simulink model "power_upfc_gto48p_mdl"  (Simulink 8.3)
settings: Solver=FixedStepDiscrete  SolverMode=SingleTasking  StartTime=0.0  StopTime=0.8  FixedStep=Ts  RelTol=1e-3
PreLoadFcn:
  | Ts=1/512/60;
undefined symbols (not defined in the file or in its folder): DiscIntNeverNeededParam
libraries: powerlib x54, powerlib_meascontrol x30, simulink_extras x2, simulink x1
(part 1 of 7)
Description:
  | Copyright 2008-2014 The MathWorks, Inc.
settings Model: Creator=MathWorks  LastModifiedBy=snt  ExtModeTrigMode=oneshot  ExtModeArmWhenConnect=off  ExtModeAutoUpdateStatusClock=off
settings DataIOCC: InitialState=xInitial_upfc  LimitDataPoints=off  SaveFinalState=on  SaveFormat=Structure  SaveOutput=off  SaveTime=off  SignalLoggingName=sigsOut
settings OptimizationCC: BlockReduction=off  BooleanDataType=off  ExpressionDepthLimit=2147483647  InitFltsAndDblsToZero=on  EfficientMapNaN2IntZero=off
settings DebuggingCC: SignalResolutionControl=TryResolveAllWithWarning  SolverPrmCheckMsg=none  MultiTaskDSMMsg=warning  MultiTaskCondExecSysMsg=none  FcnCallInpInsideContextMsg=UseLocalSettings
settings HardwareCC: TargetEndianess=LittleEndian  TargetHWDeviceType=MATLAB Host  ProdEqTarget=off
settings RTWCC: SystemTargetFile=accel.tlc  TemplateMakefile=accel_default_tmf  ProcessScript=accel_make_rtw_hook  IncludeERTFirstTime=on
settings STFCustomTargetCC: GeneratePreprocessorConditionals=Disable all  MATLABClassNameForMDSCustomization=Simulink.SoftwareTarget.TargetSpecificTriggerConfigurationBase  SystemTargetFile=accel.tlc

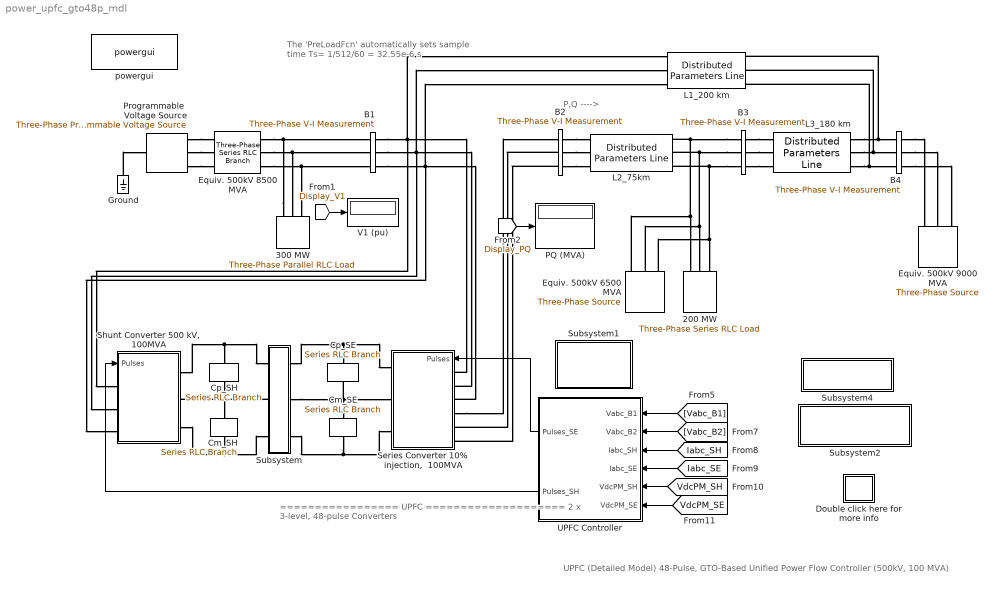
== system power_upfc_gto48p_mdl ==
  note: ================= UPFC ====================
      | 2 x   3-level, 48-pulse Converters
  note: The 'PreLoadFcn' automatically sets
      |  sample time Ts= 1/512/60 = 32.55e-6 s
  note: P,Q
      | ---->
  note: UPFC (Detailed Model)
      | 48-Pulse, GTO-Based Unified Power Flow Controller (500kV, 100 MVA)
  200 MW : powerlib/Elements/Three-Phase Series RLC Load  LConnTagsString=A|B|C  Configuration=Y (grounded)  NominalVoltage=500e3  NominalFrequency=60  ActivePower=200e6  InductivePower=0  CapacitivePower=0  Measurements=None  LoadType=constant Z
  300 MW : powerlib/Elements/Three-Phase Parallel RLC Load  LConnTagsString=A|B|C  Configuration=Y (grounded)  NominalVoltage=500e3  NominalFrequency=60  ActivePower=300e6  InductivePower=0  CapacitivePower=0  Measurements=None  LoadType=constant Z
  B1 : powerlib/Measurements/Three-Phase V-I Measurement  VoltageMeasurement=phase-to-ground  SetLabelV=on  LabelV=Vabc_B1  Vpu=on  VpuLL=off  CurrentMeasurement=yes  SetLabelI=on  LabelI=Iabc_B1  Ipu=on  Pbase=100e6  Vbase=500e3  OutputType=Magnitude  PhasorSimulation=off  PSBequivalent=0
  B2 : powerlib/Measurements/Three-Phase V-I Measurement  VoltageMeasurement=phase-to-ground  SetLabelV=on  LabelV=Vabc_B2  Vpu=on  VpuLL=off  CurrentMeasurement=yes  SetLabelI=on  LabelI=Iabc_B2  Ipu=on  Pbase=100e6  Vbase=500e3  OutputType=Magnitude  PhasorSimulation=off  PSBequivalent=0
  B3 : powerlib/Measurements/Three-Phase V-I Measurement  VoltageMeasurement=phase-to-ground  SetLabelV=on  LabelV=Vabc_B3  Vpu=on  VpuLL=off  CurrentMeasurement=yes  SetLabelI=on  LabelI=Iabc_B3  Ipu=on  Pbase=100e6  Vbase=500e3  OutputType=Magnitude  PhasorSimulation=off  PSBequivalent=0
  B4 : powerlib/Measurements/Three-Phase V-I Measurement  VoltageMeasurement=phase-to-ground  SetLabelV=on  LabelV=Vabc_B4  Vpu=on  VpuLL=off  CurrentMeasurement=no  SetLabelI=on  LabelI=Iabc_B4  Ipu=on  Pbase=100e6  Vbase=500e3  OutputType=Magnitude  PhasorSimulation=off  PSBequivalent=0
  Cm_SE : powerlib/Elements/Series RLC Branch  LConnTagsString=__new0  RConnTagsString=__new0  BranchType=C  Resistance=1.0  Inductance=1.0  SetiL0=off  InitialCurrent=0  Capacitance=2500e-6  Setx0=off  InitialVoltage=0  Measurements=Branch voltage
  Cm_SH : powerlib/Elements/Series RLC Branch  LConnTagsString=__new0  RConnTagsString=__new0  BranchType=C  Resistance=1.0  Inductance=1.0  SetiL0=off  InitialCurrent=0  Capacitance=2500e-6  Setx0=off  InitialVoltage=0  Measurements=Branch voltage
  Cp_SE : powerlib/Elements/Series RLC Branch  LConnTagsString=__new0  RConnTagsString=__new0  BranchType=C  Resistance=1.0  Inductance=1.0  SetiL0=off  InitialCurrent=0  Capacitance=2500e-6  Setx0=off  InitialVoltage=0  Measurements=Branch voltage
  Cp_SH : powerlib/Elements/Series RLC Branch  LConnTagsString=__new0  RConnTagsString=__new0  BranchType=C  Resistance=1.0  Inductance=1.0  SetiL0=off  InitialCurrent=0  Capacitance=2500e-6  Setx0=off  InitialVoltage=0  Measurements=Branch voltage
  Double click here for more info : Subsystem
      settings: OpenFcn=showdemo(bdroot(gcb))
      mask Display: disp('?')
  Equiv. 500kV 6500 MVA : powerlib/Electrical Sources/Three-Phase Source  Voltage=500e3*1.00  PhaseAngle=9.2-20  Frequency=60  InternalConnection=Yg  SpecifyImpedance=on  Resistance=0.8929  Inductance=16.58e-3  ShortCircuitLevel=6500e6  BaseVoltage=500e3  XRratio=8  BusType=swing  Pref=0  Qref=0  Qmin=-inf  Qmax=inf
  "Equiv. 500kV 8500 MVA " : powerlib/Elements/Three-Phase Series RLC Branch  LConnTagsString=A|B|C  RConnTagsString=A|B|C  BranchType=RL  Resistance=500e3^2/8500e6/10  Inductance=500e3^2/8500e6/(2*pi*60)  Capacitance=1.0  Measurements=None
  Equiv. 500kV 9000 MVA : powerlib/Electrical Sources/Three-Phase Source  Voltage=500e3*0.98  PhaseAngle=9.2-40  Frequency=60  InternalConnection=Yg  SpecifyImpedance=on  Resistance=0.8929  Inductance=16.58e-3  ShortCircuitLevel=9000e6  BaseVoltage=500e3  XRratio=10  BusType=swing  Pref=0  Qref=0  Qmin=-inf  Qmax=inf
  Ground : powerlib/Elements/Ground  LConnTagsString=a
  L1_200 km : powerlib/Elements/Distributed Parameters Line  Phases=3  Frequency=60  Resistance=[0.01273*2 0.3864]  Inductance="[0.9337e-3  4.1264e-3]"  Capacitance=[12.74e-9 7.751e-9]  Length=200  x1=[-0.00113932291666667 -5.83775963632197e-11 4414.79498015266 -499890.552538387;-0.00110677083333333 -5.5951515746169e-11 10548.8886083546 -499798.73537353;-0.00107421875 -5.35170090366527e-11 16681.393612734 -499631.650357529;-0.00104166666666667 -5.10744428624266e-11 22811.3864605943 -499389.322652774;-0.00100911458333333 -4.86241850649719e-11 28937.9439975605 -499071.788752926;-0.0009765625 -4.61666046441002e-11 35060.1435866028 -498679.096477422;-0.000944010416666667 -4.37020717023833e-11 41177.0632469823 -498211.304964274;-0.000911458333333333 -4.12309573894169e-11 47287.781793098 -497668.484661164;-0.00087890625 -3.8753633845927e-11 53391.3789732137 -497050.717314833;-0.000846354166666667 -3.62704741477269e-11 59486.935608045 -496358.09595877;-0.000813802083333333 -3.37818522495335e-11 65573.5337291839 -495590.724899204;-0.00078125 -3.12881429286507e-11 71650.2567173415 -494748.719699394;-0.000748697916666667 -2.87897217285297e-11 77716.1894403879 -493832.207162227;-0.000716145833333333 -2.62869649022133e-11 83770.4183911672 -492841.325311119;-0.00068359375 -2.37802493556737e-11 89812.0318250686 -491776.223369231;-0.000651041666666667 -2.12699525910518e-11 95840.1198973318 -490637.061736999;-0.000618489583333333 -1.87564526498067e-11 101853.774800066 -489424.011967975;-0.0005859375 -1.62401280557842e-11 107852.090898963 -488137.256742991;-0.000553385416666667 -1.37213577582123e-11 113834.164869682 -486776.989842652;-0.000520833333333333 -1.12005210746332e-11 119799.095833886 -485343.416118149;-0.00048828125 -8.67799763377903e-12 125745.985494914 -483836.751460411;-0.000455729166666667 -6.15416731840137e-12 131673.938273056 -482257.222767596;-0.000423177083333333 -3.62941020806237e-12 137582.061440429 -480605.067910913;-0.000390625 -1.10410652189606e-12 143469.465255415 -478880.535698807;-0.000358072916666667 1.42136343865122e-12 149335.263096657 -477083.885839486;-0.000325520833333333 3.94661934709283e-12 155178.571596574 -475215.388901809;-0.00029296875 6.47128090917758e-12 160998.5107744 -473275.326274544;-0.000260416666666667 8.99496792016064e-12 166794.204168703 -471263.990123986;-0.000227864583333333 1.1517300322061e-11 172564.778969376 -469181.683349959;-0.0001953125 1.40378982608969e-11 178309.366149078 -467028.719540207;-0.000162760416666667 1.65563821438901e-11 184027.100594112 -464805.422923158;-0.000130208333333333 1.90723726966315e-11 189717.121234702 -462512.128319105;-9.765625e-05 2.15854910201986e-11 195378.571174668 -460149.181089781;-6.51041666666667e-05 2.40953586482157e-11 201010.597820474 -457716.937086347;-3.25520833333333e-05 2.66015976038501e-11 206612.353009623 -455215.762595802]  x2=[-0.00113932291666667 2.86811510446065e-11 -126400.807658291 -476001.468702008;-0.00110677083333333 2.96258624700446e-11 -120550.019662708 -477516.759017374;-0.00107421875 3.05661123495671e-11 -114681.077277582 -478960.137065278;-0.00104166666666667 3.15017590850008e-11 -108794.864344047 -480331.385478293;-0.00100911458333333 3.24326617713888e-11 -102892.267304122 -481630.297751453;-0.0009765625 3.33586802182108e-11 -96974.1750672081 -482856.678273348;-0.000944010416666667 3.42796749704948e-11 -91041.4788762282 -484010.34235558;-0.000911458333333333 3.51955073298188e-11 -85095.0721734063 -485091.116260584;-0.00087890625 3.61060393751982e-11 -79135.8504657195 -486098.837227784;-0.000846354166666667 3.70111339838561e-11 -73164.7111900369 -487033.35349811;-0.000813802083333333 3.79106548518737e-11 -67182.5535779702 -487894.524336849;-0.00078125 3.8804466514717e-11 -61190.2785204514 -488682.220054839;-0.000748697916666667 3.96924343676372e-11 -55188.788432063 -489396.322028004;-0.000716145833333333 4.05744246859419e-11 -49178.9871151371 -490036.722715212;-0.00068359375 4.14503046451333e-11 -43161.7796236462 -490603.325674476;-0.000651041666666667 4.23199423409114e-11 -37138.0721269054 -491096.045577475;-0.000618489583333333 4.31832068090379e-11 -31108.7717731069 -491514.808222403;-0.0005859375 4.40399680450593e-11 -25074.7865527064 -491859.550545146;-0.000553385416666667 4.48900970238848e-11 -19037.0251616834 -492130.220628778;-0.000520833333333333 4.57334657192173e-11 -12996.3968646947 -492326.777711381;-0.00048828125 4.65699471228334e-11 -6953.81135814272 -492449.192192181;-0.000455729166666667 4.73994152637105e-11 -910.178633178308 -492497.445636008;-0.000423177083333333 4.82217452269977e-11 5133.59116134036 -492471.530776069;-0.000390625 4.90368131728272e-11 11176.587855913 -492371.451515048;-0.000358072916666667 4.98444963549644e-11 17217.9013974652 -492197.222924514;-0.000325520833333333 5.06446731392931e-11 23256.6219863994 -491948.871242651;-0.00029296875 5.14372230221327e-11 29291.840213607 -491626.433870309;-0.000260416666666667 5.22220266483862e-11 35322.6471974223 -491229.95936537;-0.000227864583333333 5.29989658295141e-11 41348.1347204965 -490759.507435436;-0.0001953125 5.37679235613336e-11 47367.3953665723 -490215.148928838;-0.000162760416666667 5.45287840416388e-11 53379.5226571368 -489596.965823965;-0.000130208333333333 5.52814326876399e-11 59383.6111879345 -488905.051216917;-9.765625e-05 5.60257561532193e-11 65378.7567653173 -488139.509307491;-6.51041666666667e-05 5.6761642346001e-11 71364.0565424133 -487300.455383481;-3.25520833333333e-05 5.74889804442311e-11 77338.6091550916 -486388.015803322]  x3=[-0.00113932291666667 8.8939155316367e-13 -16.9421274649171 53.6415754395801;-0.00110677083333333 8.87638250739574e-13 -17.5991164005912 53.4296303617768;-0.00107421875 8.85751273259906e-13 -18.2534549740699 53.2096389781707;-0.00104166666666667 8.83730904896535e-13 -18.9050446443711 52.9816344186549;-0.00100911458333333 8.81577449909503e-13 -19.5537872844871 52.7456510198774;-0.0009765625 8.79291232601213e-13 -20.1995851961625 52.50172432007;-0.000944010416666667 8.76872597267579e-13 -20.8423411246073 52.2498910536966;-0.000911458333333333 8.74321908146188e-13 -21.4819582731428 51.9901891459207;-0.00087890625 8.71639549361439e-13 -22.1183403177793 51.7226577068943;-0.000846354166666667 8.68825924866699e-13 -22.7513914217216 51.4473370258682;-0.000813802083333333 8.65881458383466e-13 -23.3810162498019 51.1642685651242;-0.00078125 8.62806593337563e-13 -24.0071199828372 50.8734949537312;-0.000748697916666667 8.59601792792356e-13 -24.6296083319082 50.5750599811256;-0.000716145833333333 8.56267539379018e-13 -25.2483875525592 50.2690085905166;-0.00068359375 8.52804335223849e-13 -25.8633644589156 49.9553868721178;-0.000651041666666667 8.49212701872656e-13 -26.4744464377175 49.6342420562063;-0.000618489583333333 8.45493180212211e-13 -27.0815414622666 49.3056225060104;-0.0005859375 8.41646330388795e-13 -27.6845581062851 48.9695777104253;-0.000553385416666667 8.3767273172384e-13 -28.2834055576847 48.6261582765613;-0.000520833333333333 8.3357298262669e-13 -28.8779936322418 48.2754159221219;-0.00048828125 8.29347700504479e-13 -29.4682327871795 47.9174034676156;-0.000455729166666667 8.24997521669153e-13 -30.0540341346521 47.5521748284011;-0.000423177083333333 8.20523101241642e-13 -30.6353094551315 47.1797850065681;-0.000390625 8.15925113053206e-13 -31.2119712106925 46.8002900826541;-0.000358072916666667 8.11204249543953e-13 -31.7839325581957 46.4137472071985;-0.000325520833333333 8.06361221658561e-13 -32.3511073623662 46.0202145921368;-0.00029296875 8.01396758739218e-13 -32.9134102087647 45.6197515020331;-0.000260416666666667 7.96311608415778e-13 -33.4707564166508 45.2124182451558;-0.000227864583333333 7.91106536493174e-13 -34.0230620517356 44.7982761643952;-0.0001953125 7.85782326836093e-13 -34.5702439388221 44.3773876280252;-0.000162760416666667 7.80339781250925e-13 -35.1122196743308 43.9498160203113;-0.000130208333333333 7.74779719365016e-13 -35.6489076387094 43.5156257319649;-9.765625e-05 7.69102978503235e-13 -36.1802270087246 43.0748821504463;-6.51041666666667e-05 7.63310413561874e-13 -36.7060977696336 42.6276516501176;-3.25520833333333e-05 7.57402896879907e-13 -37.2264407272341 42.1740015822474]  x4=[-0.00113932291666667 -7.78110289086618e-14 -894.269601115784 -3549.34214309645;-0.00110677083333333 -8.84298125759026e-14 -850.646376261383 -3560.04894780867;-0.00107421875 -9.90352790386398e-14 -806.895047191642 -3570.21962224425;-0.00104166666666667 -1.09625831152634e-13 -763.022202695786 -3579.85263473701;-0.00100911458333333 -1.20199874019693e-13 -719.03444986282 -3588.94653459072;-0.0009765625 -1.30755815227854e-13 -674.938413086522 -3597.4999522975;-0.000944010416666667 -1.41292065091199e-13 -630.740733067831 -3605.51159974411;-0.000911458333333333 -1.51807036889254e-13 -586.448065814787 -3612.98027040591;-0.00087890625 -1.62299147105944e-13 -542.067081640158 -3619.90483952857;-0.000846354166666667 -1.72766815668064e-13 -497.604464156912 -3626.28426429746;-0.000813802083333333 -1.8320846618323e-13 -453.066909271698 -3632.11758399467;-0.00078125 -1.93622526177282e-13 -408.461124176458 -3637.4039201437;-0.000748697916666667 -2.04007427331092e-13 -363.793826338355 -3642.14247664179;-0.000716145833333333 -2.14361605716744e-13 -319.071742488145 -3646.33253987974;-0.00068359375 -2.24683502033059e-13 -274.301607607154 -3649.97347884946;-0.000651041666666667 -2.34971561840418e-13 -229.490163913018 -3653.06474523891;-0.000618489583333333 -2.45224235794858e-13 -184.644159844328 -3655.60587351476;-0.0005859375 -2.55439979881393e-13 -139.77034904434 -3657.59648099244;-0.000553385416666667 -2.6561725564654e-13 -94.8754893439011 -3659.03626789378;-0.000520833333333333 -2.75754530430003e-13 -49.9663417437469 -3659.92501739216;-0.00048828125 -2.85850277595489e-13 -5.04966939631697 -3660.26259564519;-0.000455729166666667 -2.95902976760608e-13 39.8677634127502 -3660.04895181482;-0.000423177083333333 -3.05911114025844e-13 84.7791922832924 -3659.28411807502;-0.000390625 -3.15873182202538e-13 129.677853719319 -3657.96820960694;-0.000358072916666667 -3.25787681039864e-13 174.556986147568 -3656.10142458156;-0.000325520833333333 -3.35653117450768e-13 219.409830935775 -3653.68404412984;-0.00029296875 -3.45468005736812e-13 264.229633410495 -3650.71643230038;-0.000260416666666667 -3.55230867811923e-13 309.009643874337 -3647.1990360046;-0.000227864583333333 -3.64940233424984e-13 353.743118622438 -3643.13238494946;-0.0001953125 -3.74594640381247e-13 398.423320958044 -3638.51709155763;-0.000162760416666667 -3.84192634762536e-13 443.043522207029 -3633.35385087534;-0.000130208333333333 -3.93732771146201e-13 487.597002731213 -3627.64344046763;-9.765625e-05 -4.03213612822794e-13 532.077052940308 -3621.3867203013;-6.51041666666667e-05 -4.12633732012433e-13 576.476974302363 -3614.58463261541;-3.25520833333333e-05 -4.21991710079816e-13 620.790080352538 -3607.23820177933]  x5=0.00113108313399149  V1=ones(3,3)  V2=ones(3,3)  I1=ones(3,3)  I2=ones(3,3)  nHarmo=1  Measurements=None
      settings: AttributesFormatString=\n
  L2_75km : powerlib/Elements/Distributed Parameters Line  Phases=3  Frequency=60  Resistance=[0.01273*2 0.3864]  Inductance="[0.9337e-3  4.1264e-3]"  Capacitance=[12.74e-9 7.751e-9]  Length=75  x1=[-0.000455729166666667 -1.27140528390199e-10 0 0;-0.000423177083333333 -1.26495463510687e-10 0 0;-0.000390625 -1.25831348879657e-10 0 0;-0.000358072916666667 -1.25148284510329e-10 0 0;-0.000325520833333333 -1.24446373269686e-10 0 0;-0.00029296875 -1.23725720862978e-10 0 0;-0.000260416666666667 -1.22986435817807e-10 166794.132131736 -471263.82102114;-0.000227864583333333 -1.22228629467782e-10 172564.704862681 -469181.515143851;-0.0001953125 -1.21452415935751e-10 178309.289983816 -467028.552256167;-0.000162760416666667 -1.20657912116618e-10 184027.022381753 -464805.256586379;-0.000130208333333333 -1.19845237659734e-10 189717.040987023 -462511.962954638;-9.765625e-05 -1.19014514950884e-10 195378.488903755 -460149.016722528;-6.51041666666667e-05 -1.18165869093852e-10 201010.513538717 -457716.77374106;-3.25520833333333e-05 -1.17299427891583e-10 206612.266729715 -455215.600297082]  x2=[-0.000455729166666667 -2.36997076318553e-11 0 0;-0.000423177083333333 -2.41108726134989e-11 0 0;-0.000390625 -2.45184065864136e-11 0 0;-0.000358072916666667 -2.49222481774822e-11 0 0;-0.000325520833333333 -2.53223365696465e-11 0 0;-0.00029296875 -2.57186115110664e-11 0 0;-0.000260416666666667 -2.61110133241931e-11 120220.444766576 -484737.668130302;-0.000227864583333333 -2.6499482914757e-11 126159.86924118 -483225.878484715;-0.0001953125 -2.68839617806668e-11 132080.294503528 -481641.316799273;-0.000162760416666667 -2.72643920208194e-11 137980.828959354 -479984.221703137;-0.000130208333333333 -2.76407163438199e-11 143860.584009871 -478254.842748733;-9.765625e-05 -2.80128780766097e-11 149718.674185598 -476453.440374171;-6.51041666666667e-05 -2.83808211730005e-11 155554.2172797 -474580.285864021;-3.25520833333333e-05 -2.87444902221156e-11 161366.334480854 -472635.661308464]  x3=[-0.000455729166666667 1.80871262636325e-13 0 0;-0.000423177083333333 1.68315951242698e-13 0 0;-0.000390625 1.55735292085928e-13 0 0;-0.000358072916666667 1.43131179767009e-13 0 0;-0.000325520833333333 1.30505512418895e-13 0 0;-0.00029296875 1.17860191420648e-13 0 0;-0.000260416666666667 1.05197121111097e-13 -104.968306035297 -46.5279101834584;-0.000227864583333333 9.25182085020516e-14 -104.389433083734 -47.8125293036924;-0.0001953125 7.98253629911147e-14 -103.794839467522 -49.0899480328816;-0.000162760416666667 6.71204960741322e-14 -103.184614730275 -50.3599739964641;-0.000130208333333333 5.44055210573295e-14 -102.558850769592 -51.6224159332012;-9.765625e-05 4.16823527691748e-14 -101.917641823224 -52.877083723981;-6.51041666666667e-05 2.89529072720129e-14 -101.26108445488 -54.1237884204491;-3.25520833333333e-05 1.62191015735129e-14 -100.589277539684 -55.362342273464]  x4=[-0.000455729166666667 -2.77784366561629e-13 0 0;-0.000423177083333333 -3.06117246189209e-13 0 0;-0.000390625 -3.34404025685501e-13 0 0;-0.000358072916666667 -3.6264044516556e-13 0 0;-0.000325520833333333 -3.90822252328473e-13 0 0;-0.00029296875 -4.18945203097742e-13 0 0;-0.000260416666666667 -4.47005062260427e-13 987.851977766537 -3517.72393741717;-0.000227864583333333 -4.74997604104949e-13 1030.94547830602 -3505.3365959085;-0.0001953125 -5.02918613057471e-13 1073.88372224859 -3492.42136360213;-0.000162760416666667 -5.30763884316747e-13 1116.66024325264 -3478.98018548453;-0.000130208333333333 -5.58529224487347e-13 1159.26859933146 -3465.01508574769;-9.765625e-05 -5.86210452211172e-13 1201.70237382334 -3450.52816748427;-6.51041666666667e-05 -6.13803398797145e-13 1243.95517635794 -3435.52161237087;-3.25520833333333e-05 -6.41303908849006e-13 1286.0206438186 -3419.99768033948]  x5=0.000424156175246807  V1=ones(3,3)  V2=ones(3,3)  I1=ones(3,3)  I2=ones(3,3)  nHarmo=1  Measurements=None
      settings: AttributesFormatString=\n
  L3_180 km : powerlib/Elements/Distributed Parameters Line  Phases=3  Frequency=60  Resistance=[0.01273*2 0.3864]  Inductance="[0.9337e-3  4.1264e-3]"  Capacitance=[12.74e-9 7.751e-9]  Length=180  x1=[-0.00104166666666667 -2.13196564095776e-11 0 0;-0.00100911458333333 -2.16197072149166e-11 0 0;-0.0009765625 -2.19165021718726e-11 0 0;-0.000944010416666667 -2.22099965842166e-11 0 0;-0.000911458333333333 -2.25001462527699e-11 0 0;-0.00087890625 -2.27869074820596e-11 0 0;-0.000846354166666667 -2.30702370868993e-11 0 0;-0.000813802083333333 -2.33500923988927e-11 0 0;-0.00078125 -2.36264312728593e-11 0 0;-0.000748697916666667 -2.3899212093181e-11 0 0;-0.000716145833333333 -2.41683937800696e-11 0 0;-0.00068359375 -2.44339357957533e-11 0 0;-0.000651041666666667 -2.46957981505813e-11 47793.4519494708 -497131.117709433;-0.000618489583333333 -2.49539414090461e-11 53890.4167344322 -496507.185475161;-0.0005859375 -2.52083266957225e-11 59979.2658208578 -495808.481085053;-0.000553385416666667 -2.5458915701122e-11 66059.0822504719 -495035.109761421;-0.000520833333333333 -2.57056706874622e-11 72128.9504252835 -494187.187971141;-0.00048828125 -2.59485544943497e-11 78187.9562454721 -493264.843408115;-0.000455729166666667 -2.61875305443767e-11 84235.1872470481 -492268.214974044;-0.000423177083333333 -2.6422562848629e-11 90269.7327392661 -491197.452757502;-0.000390625 -2.66536160121061e-11 96290.6839417717 -490052.71801134;-0.000358072916666667 -2.68806552390515e-11 102297.134121461 -488834.183128402;-0.000325520833333333 -2.71036463381927e-11 108288.178729029 -487542.031615558;-0.00029296875 -2.73225557278904e-11 114262.915535197 -486176.458066074;-0.000260416666666667 -2.75373504411958e-11 120220.444766576 -484737.668130302;-0.000227864583333333 -2.7747998130815e-11 126159.86924118 -483225.878484715;-0.0001953125 -2.7954467073981e-11 132080.294503528 -481641.316799273;-0.000162760416666667 -2.81567261772302e-11 137980.828959354 -479984.221703137;-0.000130208333333333 -2.83547449810856e-11 143860.584009871 -478254.842748733;-9.765625e-05 -2.85484936646439e-11 149718.674185598 -476453.440374171;-6.51041666666667e-05 -2.87379430500659e-11 155554.2172797 -474580.285864021;-3.25520833333333e-05 -2.8923064606971e-11 161366.334480854 -472635.661308464]  x2=[-0.00104166666666667 3.15017590850008e-11 0 0;-0.00100911458333333 3.24326617713888e-11 0 0;-0.0009765625 3.33586802182108e-11 0 0;-0.000944010416666667 3.42796749704948e-11 0 0;-0.000911458333333333 3.51955073298188e-11 0 0;-0.00087890625 3.61060393751982e-11 0 0;-0.000846354166666667 3.70111339838561e-11 0 0;-0.000813802083333333 3.79106548518737e-11 0 0;-0.00078125 3.8804466514717e-11 0 0;-0.000748697916666667 3.96924343676372e-11 0 0;-0.000716145833333333 4.05744246859419e-11 0 0;-0.00068359375 4.14503046451333e-11 0 0;-0.000651041666666667 4.23199423409114e-11 -37138.0721269054 -491096.045577475;-0.000618489583333333 4.31832068090379e-11 -31108.7717731069 -491514.808222403;-0.0005859375 4.40399680450593e-11 -25074.7865527064 -491859.550545146;-0.000553385416666667 4.48900970238848e-11 -19037.0251616834 -492130.220628778;-0.000520833333333333 4.57334657192173e-11 -12996.3968646947 -492326.777711381;-0.00048828125 4.65699471228334e-11 -6953.81135814272 -492449.192192181;-0.000455729166666667 4.73994152637105e-11 -910.178633178308 -492497.445636008;-0.000423177083333333 4.82217452269977e-11 5133.59116134036 -492471.530776069;-0.000390625 4.90368131728272e-11 11176.587855913 -492371.451515048;-0.000358072916666667 4.98444963549644e-11 17217.9013974652 -492197.222924514;-0.000325520833333333 5.06446731392931e-11 23256.6219863994 -491948.871242651;-0.00029296875 5.14372230221327e-11 29291.840213607 -491626.433870309;-0.000260416666666667 5.22220266483862e-11 35322.6471974223 -491229.95936537;-0.000227864583333333 5.29989658295141e-11 41348.1347204965 -490759.507435436;-0.0001953125 5.37679235613336e-11 47367.3953665723 -490215.148928838;-0.000162760416666667 5.45287840416388e-11 53379.5226571368 -489596.965823965;-0.000130208333333333 5.52814326876399e-11 59383.6111879345 -488905.051216917;-9.765625e-05 5.60257561532193e-11 65378.7567653173 -488139.509307491;-6.51041666666667e-05 5.6761642346001e-11 71364.0565424133 -487300.455383481;-3.25520833333333e-05 5.74889804442311e-11 77338.6091550916 -486388.015803322]  x3=[-0.00104166666666667 1.7095544161851e-13 0 0;-0.00100911458333333 1.71091661173283e-13 0 0;-0.0009765625 1.71202114953208e-13 0 0;-0.000944010416666667 1.71286786324352e-13 0 0;-0.000911458333333333 1.71345662535518e-13 0 0;-0.00087890625 1.71378734720164e-13 0 0;-0.000846354166666667 1.71385997897743e-13 0 0;-0.000813802083333333 1.71367450974445e-13 0 0;-0.00078125 1.71323096743369e-13 0 0;-0.000748697916666667 1.712529418841e-13 0 0;-0.000716145833333333 1.71156996961701e-13 0 0;-0.00068359375 1.71035276425125e-13 0 0;-0.000651041666666667 1.70887798605035e-13 -40.3366356617392 -492.38414570646;-0.000618489583333333 1.70714585711051e-13 -34.2912874919405 -492.842062654694;-0.0005859375 1.70515663828396e-13 -28.2407751803788 -493.225759401108;-0.000553385416666667 1.70291062913975e-13 -22.1860099119526 -493.535178162383;-0.000520833333333333 1.70040816791859e-13 -16.1279035120403 -493.770272341191;-0.00048828125 1.69764963148193e-13 -10.0673683091821 -493.931006533215;-0.000455729166666667 1.69463543525521e-13 -4.0053169976873 -494.017356532477;-0.000423177083333333 1.6913660331653e-13 2.05733749981469 -494.029309334983;-0.000390625 1.68784191757214e-13 8.11968216985667 -493.966863140685;-0.000358072916666667 1.68406361919455e-13 14.1808040456304 -493.830027353752;-0.000325520833333333 1.68003170703039e-13 20.239790344476 -493.618822581149;-0.00029296875 1.67574678827079e-13 26.2957286053435 -493.333280629538;-0.000260416666666667 1.67120950820876e-13 32.3477068262063 -492.973444500486;-0.000227864583333333 1.66642055014199e-13 38.3948136014053 -492.539368383992;-0.0001953125 1.66138063526994e-13 44.4361382589031 -492.031117650321;-0.000162760416666667 1.65609052258526e-13 50.4707709974282 -491.448768840164;-0.000130208333333333 1.65055100875945e-13 56.4978030234871 -490.792409653111;-9.765625e-05 1.64476292802293e-13 62.5163266882259 -490.062138934441;-6.51041666666667e-05 1.63872715203936e-13 68.5254356241186 -489.258066660237;-3.25520833333333e-05 1.63244458977441e-13 74.5242248814626 -488.380313920827]  x4=[-0.00104166666666667 7.63530042489158e-13 0 0;-0.00100911458333333 7.54755688850395e-13 0 0;-0.0009765625 7.45867671781101e-13 0 0;-0.000944010416666667 7.36867329783954e-13 0 0;-0.000911458333333333 7.27756018277352e-13 0 0;-0.00087890625 7.18535109391295e-13 0 0;-0.000846354166666667 7.09205991760743e-13 0 0;-0.000813802083333333 6.99770070316497e-13 0 0;-0.00078125 6.90228766073618e-13 0 0;-0.000748697916666667 6.80583515917429e-13 0 0;-0.000716145833333333 6.70835772387125e-13 0 0;-0.00068359375 6.60987003457028e-13 0 0;-0.000651041666666667 6.51038692315512e-13 -346.315027735524 -3116.34913325067;-0.000618489583333333 6.40992337141642e-13 -308.046553150504 -3120.36429601412;-0.0005859375 6.30849450879553e-13 -269.731687887663 -3123.90954339221;-0.000553385416666667 6.20611561010608e-13 -231.376202024777 -3126.9843414837;-0.000520833333333333 6.10280209323364e-13 -192.985871756935 -3129.58822723531;-0.00048828125 5.99856951681383e-13 -154.566478526664 -3131.72080851143;-0.000455729166666667 5.89343357788926e-13 -116.123808153267 -3133.38176415317;-0.000423177083333333 5.78741010954561e-13 -77.6636499614995 -3134.5708440267;-0.000390625 5.68051507852723e-13 -39.1917959097169 -3135.28786906099;-0.000358072916666667 5.5727645828326e-13 -0.714039717629134 -3135.53273127469;-0.000325520833333333 5.46417484929004e-13 37.7638240062137 -3135.30539379245;-0.00029296875 5.35476223111399e-13 76.2360006370674 -3134.60589085047;-0.000260416666666667 5.24454320544229e-13 114.696696406643 -3133.43432779132;-0.000227864583333333 5.1335343708548e-13 153.140119275628 -3131.79088104807;-0.0001953125 5.02175244487369e-13 191.560479805943 -3129.67579811778;-0.000162760416666667 4.90921426144583e-13 229.951992032615 -3127.08939752414;-0.000130208333333333 4.79593676840771e-13 268.308874335116 -3124.03206876957;-9.765625e-05 4.68193702493311e-13 306.62535030806 -3120.50427227653;-6.51041666666667e-05 4.56723219896407e-13 344.895649631104 -3116.50653931821;-3.25520833333333e-05 4.45183956462547e-13 383.11400893794 -3112.03947193848]  x5=0.00101797482059234  V1=ones(3,3)  V2=ones(3,3)  I1=ones(3,3)  I2=ones(3,3)  nHarmo=1  Measurements=None
      settings: AttributesFormatString=\n
  PQ (MVA) : Display
      settings: Format=bank  SampleTime=Ts*100
  Programmable  Voltage Source : powerlib/Electrical Sources/Three-Phase Programmable Voltage Source  PositiveSequence="[500e3*1.0491 9.2  60]"  VariationEntity=None  VariationType=Modulation  VariationTypeAlt=Step  VariationStep=-0.3  VariationRate=0.5  VariationMagnitude=0.4  VariationFrequency=2  VariationTiming=[0.1 1.2]  VariationPhaseA=off  Amplitudes="[1  0.8  1.2  1.0 ]"  TimeValues=[0 0.1 0.25 0.4]  HarmonicGeneration=off  HarmonicA=[3 0.2 -25 0]  HarmonicB="[2 0.15  35 2]"  Timing="[0.1  0.6]"  BusType=swing  Pref=0  Qref=0  Qmin=-inf  Qmax=inf
  "Series Converter 10% injection,  100MVA" : Subsystem
  "Shunt Converter 500 kV, 100MVA" : Subsystem
  Subsystem : Subsystem
      mask Display: disp('Sw')
  Subsystem1 : Subsystem  mask(UPFC GUI){OpMode=UPFC  (Power Flow Control), Par_VarControl=[0.3  0.5  +0.8  -0.8 ], Par_Vref=[ 1  1.005  0.3 *100], Par_SSSC=[ 0.0  0.08  0.3  ], Par_UPFC_Pref=[  +8.7  +10   0.25  ], Par_UPFC_Qref=[  -0.6  +0.7  0.5  ]}
      mask prompts: OpMode "Operation Mode:"; Par_VarControl "STATCOM (Qref): [T1 T2 Q1 Q2]"; Par_Vref "STATCOM Vref (pu): [ Initial   Final  StepTime ]"; Par_SSSC "SSSC Votage Injection (pu): [ Initial  Final  StepTime ]"; Par_UPFC_Pref "UPFC Pref (pu): [ Initial  Final  StepTime ]"; Par_UPFC_Qref "UPFC Qref (pu): [ Initial  Final  StepTime ]"
      mask TypeOptions OpMode: STATCOM (Var Control) | STATCOM (Voltage Control) | SSSC (Voltage Injection) | STATCOM  (Voltage Control) + SSSC (Voltage Injection) | UPFC  (Power Flow Control)
      mask Display: disp('UPFC\nGUI')
  Subsystem2 : Subsystem  mask(UPFC GUI){OpMode=SSSC (Voltage Injection), Par_VarControl=[0.05 0.15 -0.5 0.5]*100, Par_Vref=[ 1  1.005  0.1*100 ], Par_SSSC=[ 0.0  0.08 0.1*100 ], Par_UPFC_Pref=[  8.7  10  0.1*100 ], Par_UPFC_Qref=[  -0.6  +0.5  0.1*100 ]}
      mask prompts: OpMode "Operation Mode:"; Par_VarControl "STATCOM (Qref): [T1 T2 Q1 Q2]"; Par_Vref "STATCOM Vref (pu): [ Initial   Final  StepTime ]"; Par_SSSC "SSSC Votage Injection (pu): [ Initial  Final  StepTime ]"; Par_UPFC_Pref "UPFC Pref (pu): [ Initial  Final  StepTime ]"; Par_UPFC_Qref "UPFC Qref (pu): [ Initial  Final  StepTime ]"
      settings: OpenFcn=openfig('power_upfc_gto48p_PQregion.fig');
      mask TypeOptions OpMode: STATCOM (Var Control) | STATCOM (Voltage Control) | SSSC (Voltage Injection) | STATCOM  (Voltage Control) + SSSC (Voltage Injection) | UPFC  (Power Flow Control)
      mask Display: disp('Show UPFC\nControllable Region')
  Subsystem4 : Subsystem
      mask Display: disp('Show Scopes')
  UPFC Controller : Subsystem
  V1 (pu) : Display
      settings: Format=bank  SampleTime=Ts*100
  powergui : powerlib/powergui  Priority=2  SimulationMode=Discrete  SolverType=Tustin  SampleTime=Ts  frequency=60  SPID=off  DisableSnubberDevices=off  DisableRonSwitches=off  DisableVfSwitches=off  SwTol=0  Interpol=off  DisplayEquations=off  Ts=0  methode=off  frequencyindice=60  Pbase=100e6  ErrMax=1e-4  Iterations=50  UnitsV=kV  UnitsW=MW  FunctionMessages=off  echomessages=off  HookPort=off  EnableUseOfTLC=off  x0status=blocks  RestoreLinks=yes  ResistiveCurrentMeasurement=off  Frange=[0:2:500]  Ylog=off  Xlog=on  ShowGrid=off  save=off  variable=ZData  structure=0  ZoomFFT=on  StartTime=0.0  cycles=1  DisplayStyle=1  fundamental=60  FreqAxis=off  MaxFrequency=1000  frequencyindicesteady=1  RmsSteady=1  display=off
  wires:
  [Vabc_B1] -> UPFC Controller/1(Vabc_B1)
  [Vabc_B2] -> UPFC Controller/2(Vabc_B2)
  [Iabc_SH] -> UPFC Controller/3("Iabc_SH ")
  [Iabc_SE] -> UPFC Controller/4(Iabc_SE)
  [VdcPM_SH] -> UPFC Controller/5("VdcPM_SH ")
  [VdcPM_SE] -> UPFC Controller/6(VdcPM_SE)
  [Display_V1] -> V1 (pu)/1
  [Display_PQ] -> PQ (MVA)/1
  UPFC Controller/2(Pulses_SH) -> "Shunt Converter 500 kV, 100MVA"/1(Pulses)
  UPFC Controller/1(Pulses_SE) -> "Series Converter 10% injection,  100MVA"/1(Pulses)
  connections:
  Ground/LConn1 -- Programmable  Voltage Source/LConn1
  Programmable  Voltage Source/RConn1 -- "Equiv. 500kV 8500 MVA "/LConn1
  Programmable  Voltage Source/RConn2 -- "Equiv. 500kV 8500 MVA "/LConn2
  Programmable  Voltage Source/RConn3 -- "Equiv. 500kV 8500 MVA "/LConn3
  Subsystem/LConn2 -- "Shunt Converter 500 kV, 100MVA"/RConn2 -- Cp_SH/RConn1 -- Cm_SH/LConn1
  Subsystem/RConn3 -- "Series Converter 10% injection,  100MVA"/RConn3 -- Cm_SE/RConn1
  Subsystem/RConn1 -- "Series Converter 10% injection,  100MVA"/RConn1 -- Cp_SE/LConn1
  B3/LConn1 -- 200 MW/LConn1 -- Equiv. 500kV 6500 MVA/RConn1 -- L2_75km/RConn1
  B3/LConn2 -- 200 MW/LConn2 -- Equiv. 500kV 6500 MVA/RConn2 -- L2_75km/RConn2
  B3/LConn3 -- 200 MW/LConn3 -- Equiv. 500kV 6500 MVA/RConn3 -- L2_75km/RConn3
  "Equiv. 500kV 8500 MVA "/RConn2 -- 300 MW/LConn2 -- B1/LConn2
  "Equiv. 500kV 8500 MVA "/RConn3 -- 300 MW/LConn3 -- B1/LConn3
  B2/RConn1 -- L2_75km/LConn1
  B2/RConn2 -- L2_75km/LConn2
  B2/RConn3 -- L2_75km/LConn3
  B3/RConn1 -- L3_180 km/LConn1
  B3/RConn2 -- L3_180 km/LConn2
  B3/RConn3 -- L3_180 km/LConn3
  300 MW/LConn1 -- "Equiv. 500kV 8500 MVA "/RConn1 -- B1/LConn1
  L3_180 km/RConn1 -- B4/LConn1 -- L1_200 km/RConn1
  L3_180 km/RConn2 -- B4/LConn2 -- L1_200 km/RConn2
  L3_180 km/RConn3 -- B4/LConn3 -- L1_200 km/RConn3
  B4/RConn1 -- Equiv. 500kV 9000 MVA/RConn1
  B4/RConn2 -- Equiv. 500kV 9000 MVA/RConn2
  B4/RConn3 -- Equiv. 500kV 9000 MVA/RConn3
  "Shunt Converter 500 kV, 100MVA"/LConn1 -- B1/RConn1 -- L1_200 km/LConn1 -- "Series Converter 10% injection,  100MVA"/LConn1
  "Series Converter 10% injection,  100MVA"/LConn2 -- B1/RConn2 -- L1_200 km/LConn2 -- "Shunt Converter 500 kV, 100MVA"/LConn2
  "Shunt Converter 500 kV, 100MVA"/LConn3 -- B1/RConn3 -- L1_200 km/LConn3 -- "Series Converter 10% injection,  100MVA"/LConn3
  "Series Converter 10% injection,  100MVA"/LConn4 -- B2/LConn1
  B2/LConn2 -- "Series Converter 10% injection,  100MVA"/LConn5
  B2/LConn3 -- "Series Converter 10% injection,  100MVA"/LConn6
  Subsystem/RConn2 -- "Series Converter 10% injection,  100MVA"/RConn2 -- Cm_SE/LConn1 -- Cp_SE/RConn1
  "Shunt Converter 500 kV, 100MVA"/RConn1 -- Subsystem/LConn1 -- Cp_SH/LConn1
  "Shunt Converter 500 kV, 100MVA"/RConn3 -- Subsystem/LConn3 -- Cm_SH/RConn1

== system power_upfc_gto48p_mdl/Double click here for more info ==

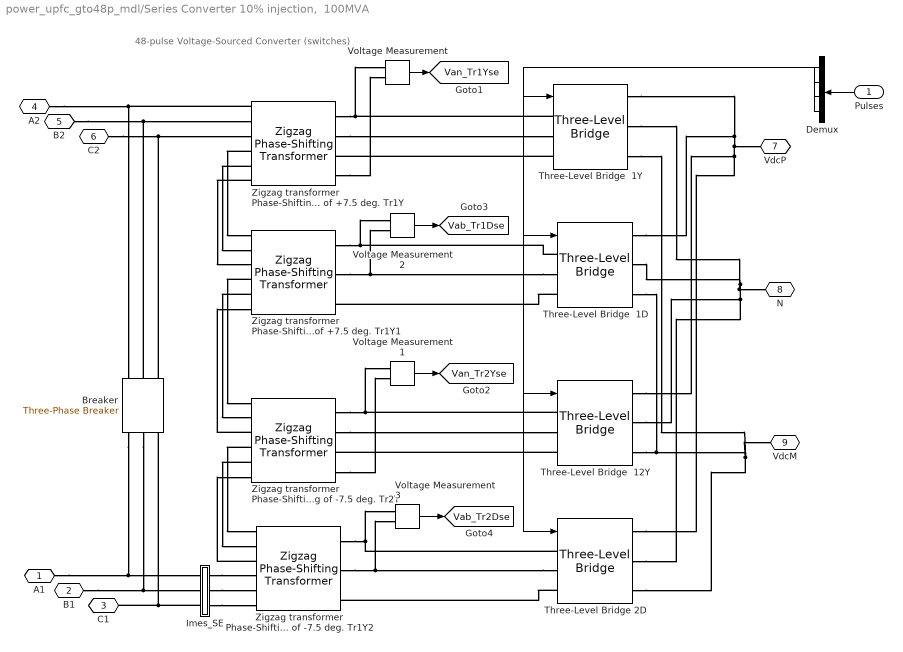
== system power_upfc_gto48p_mdl/Series Converter 10% injection,  100MVA ==
  note: 48-pulse Voltage-Sourced Converter
      | (switches)
  Pulses : Inport  PortDimensions=48
  Breaker : powerlib/Elements/Three-Phase Breaker  InitialState=closed  SwitchA=on  SwitchB=on  SwitchC=on  SwitchTimes=[ 0]  External=off  BreakerResistance=0.0001  SnubberResistance=1e6  SnubberCapacitance=inf  Measurements=None
      settings: AttributesFormatString=\n
  Demux : Demux  Outputs=[12 12 12 12]
  Imes_SE : Subsystem
  Three-Level Bridge  12Y : powerlib/Power Electronics/Three-Level Bridge  Arms=3  SnubberResistance=1e5  SbubberCapacitance=inf  Device=GTO / Diodes  Ron=1e-4  ForwardVoltages="[  0  0  ]"  Measurements=None
  Three-Level Bridge  1D : powerlib/Power Electronics/Three-Level Bridge  Arms=3  SnubberResistance=1e5  SbubberCapacitance=inf  Device=GTO / Diodes  Ron=1e-4  ForwardVoltages="[  0  0  ]"  Measurements=None
  Three-Level Bridge  1Y : powerlib/Power Electronics/Three-Level Bridge  Arms=3  SnubberResistance=1e5  SbubberCapacitance=inf  Device=GTO / Diodes  Ron=1e-4  ForwardVoltages="[  0  0  ]"  Measurements=None
  Three-Level Bridge 2D : powerlib/Power Electronics/Three-Level Bridge  Arms=3  SnubberResistance=1e5  SbubberCapacitance=inf  Device=GTO / Diodes  Ron=1e-4  ForwardVoltages="[  0  0  ]"  Measurements=None
  Voltage Measurement{,1..3} (4 alike) : powerlib/Measurements/Voltage Measurement  Tag=PoWeRsYsTeMmEaSuReMeNt  PhasorSimulation=off  OutputType=Magnitude  PSBequivalent=0
  Zigzag transformer Phase-Shifting of +7.5 deg. Tr1Y : powerlib/Elements/Zigzag Phase-Shifting Transformer  SecondaryConnection=Yn  UNITS=pu  NominalPower=[ 100e6/4 60]  PrimaryVoltage=12.5e3  SecondaryVoltage="[ 12.5e3  +7.5]"  Winding1=[ 0.05/30 0.05 ]  Winding2=[ 0.05/30 0.05 ]  Winding3=[ 0.05/30 0.05 ]  SetSaturation=off  RmLm=[ 500 500 ]  Rm=500  Saturation=[ 0,0 ; 0.0024,1.2 ; 1.0,1.52 ]  SetInitialFlux=off  Measurements=None  InitialFluxes=[0,0,0]  MoreParameters=off  BreakLoop=off  DataType=off
      settings: AttributesFormatString=\n
  Zigzag transformer Phase-Shifting of +7.5 deg. Tr1Y1 : powerlib/Elements/Zigzag Phase-Shifting Transformer  SecondaryConnection=Delta D1(-30 deg.)  UNITS=pu  NominalPower=[ 100e6/4 60]  PrimaryVoltage=12.5e3  SecondaryVoltage="[ 12.5e3  +7.5]"  Winding1=[ 0.05/30 0.05 ]  Winding2=[ 0.05/30 0.05 ]  Winding3=[ 0.05/30 0.05 ]  SetSaturation=off  RmLm=[ 500 500 ]  Rm=500  Saturation=[ 0,0 ; 0.0024,1.2 ; 1.0,1.52 ]  SetInitialFlux=off  Measurements=None  InitialFluxes=[0,0,0]  MoreParameters=off  BreakLoop=off  DataType=off
      settings: AttributesFormatString=\n
  Zigzag transformer Phase-Shifting of -7.5 deg. Tr1Y2 : powerlib/Elements/Zigzag Phase-Shifting Transformer  SecondaryConnection=Delta D1(-30 deg.)  UNITS=pu  NominalPower=[ 100e6/4 60]  PrimaryVoltage=12.5e3  SecondaryVoltage="[ 12.5e3  -7.5]"  Winding1=[ 0.05/30 0.05 ]  Winding2=[ 0.05/30 0.05 ]  Winding3=[ 0.05/30 0.05 ]  SetSaturation=off  RmLm=[ 500 500 ]  Rm=500  Saturation=[ 0,0 ; 0.0024,1.2 ; 1.0,1.52 ]  SetInitialFlux=off  Measurements=None  InitialFluxes=[0,0,0]  MoreParameters=off  BreakLoop=off  DataType=off
      settings: AttributesFormatString=\n
  Zigzag transformer Phase-Shifting of -7.5 deg. Tr2Y : powerlib/Elements/Zigzag Phase-Shifting Transformer  SecondaryConnection=Yn  UNITS=pu  NominalPower=[ 100e6/4 60]  PrimaryVoltage=12.5e3  SecondaryVoltage="[ 12.5e3  -7.5]"  Winding1=[ 0.05/30 0.05 ]  Winding2=[ 0.05/30 0.05 ]  Winding3=[ 0.05/30 0.05 ]  SetSaturation=off  RmLm=[ 500 500 ]  Rm=500  Saturation=[ 0,0 ; 0.0024,1.2 ; 1.0,1.52 ]  SetInitialFlux=off  Measurements=None  InitialFluxes=[0,0,0]  MoreParameters=off  BreakLoop=off  DataType=off
      settings: AttributesFormatString=\n
  "A1 " : PMIOPort  Port=1  Side=Left
  "B1 " : PMIOPort  Port=2  Side=Left
  C1 : PMIOPort  Port=3  Side=Left
  "A2 " : PMIOPort  Port=4  Side=Left
  "B2 " : PMIOPort  Port=5  Side=Left
  "C2 " : PMIOPort  Port=6  Side=Left
  VdcP : PMIOPort  Port=7  Side=Right
  N : PMIOPort  Port=8  Side=Right
  VdcM : PMIOPort  Port=9  Side=Right
  tag scope: Vab_Tr1Dse=global, Vab_Tr2Dse=global, Van_Tr1Yse=global, Van_Tr2Yse=global
  wires:
  Pulses/1 -> Demux/1
  Demux/4 -> Three-Level Bridge 2D/1
  Demux/3 -> Three-Level Bridge  12Y/1
  Demux/2 -> Three-Level Bridge  1D/1
  Demux/1 -> Three-Level Bridge  1Y/1
  Voltage Measurement3/1 -> [Vab_Tr2Dse]
  Voltage Measurement2/1 -> [Vab_Tr1Dse]
  Voltage Measurement1/1 -> [Van_Tr2Yse]
  Voltage Measurement/1 -> [Van_Tr1Yse]
  connections:
  Zigzag transformer Phase-Shifting of -7.5 deg. Tr2Y/RConn4 -- Voltage Measurement1/LConn2
  Zigzag transformer Phase-Shifting of +7.5 deg. Tr1Y/RConn4 -- Voltage Measurement/LConn2
  Three-Level Bridge  1Y/RConn3 -- Three-Level Bridge  1D/RConn3 -- Three-Level Bridge  12Y/RConn3 -- VdcM/RConn1 -- Three-Level Bridge 2D/RConn3
  Three-Level Bridge  12Y/RConn2 -- Three-Level Bridge  1D/RConn2 -- Three-Level Bridge  1Y/RConn2 -- N/RConn1 -- Three-Level Bridge 2D/RConn2
  Three-Level Bridge  1Y/RConn1 -- Three-Level Bridge  12Y/RConn1 -- Three-Level Bridge 2D/RConn1 -- VdcP/RConn1 -- Three-Level Bridge  1D/RConn1
  Three-Level Bridge  1D/LConn1 -- Zigzag transformer Phase-Shifting of +7.5 deg. Tr1Y1/RConn1 -- Voltage Measurement2/LConn1
  Imes_SE/RConn1 -- Zigzag transformer Phase-Shifting of -7.5 deg. Tr1Y2/LConn4
  Imes_SE/RConn2 -- Zigzag transformer Phase-Shifting of -7.5 deg. Tr1Y2/LConn5
  Imes_SE/RConn3 -- Zigzag transformer Phase-Shifting of -7.5 deg. Tr1Y2/LConn6
  "A1 "/RConn1 -- Imes_SE/LConn1 -- Breaker/RConn1
  Zigzag transformer Phase-Shifting of +7.5 deg. Tr1Y/LConn4 -- Zigzag transformer Phase-Shifting of +7.5 deg. Tr1Y1/LConn1
  Zigzag transformer Phase-Shifting of +7.5 deg. Tr1Y/LConn5 -- Zigzag transformer Phase-Shifting of +7.5 deg. Tr1Y1/LConn2
  Zigzag transformer Phase-Shifting of +7.5 deg. Tr1Y/LConn6 -- Zigzag transformer Phase-Shifting of +7.5 deg. Tr1Y1/LConn3
  Zigzag transformer Phase-Shifting of +7.5 deg. Tr1Y1/LConn4 -- Zigzag transformer Phase-Shifting of -7.5 deg. Tr2Y/LConn1
  Zigzag transformer Phase-Shifting of +7.5 deg. Tr1Y1/LConn5 -- Zigzag transformer Phase-Shifting of -7.5 deg. Tr2Y/LConn2
  Zigzag transformer Phase-Shifting of -7.5 deg. Tr2Y/LConn3 -- Zigzag transformer Phase-Shifting of +7.5 deg. Tr1Y1/LConn6
  Zigzag transformer Phase-Shifting of -7.5 deg. Tr2Y/LConn4 -- Zigzag transformer Phase-Shifting of -7.5 deg. Tr1Y2/LConn1
  Zigzag transformer Phase-Shifting of -7.5 deg. Tr2Y/LConn5 -- Zigzag transformer Phase-Shifting of -7.5 deg. Tr1Y2/LConn2
  Zigzag transformer Phase-Shifting of -7.5 deg. Tr1Y2/LConn3 -- Zigzag transformer Phase-Shifting of -7.5 deg. Tr2Y/LConn6
  Three-Level Bridge  1Y/LConn1 -- Zigzag transformer Phase-Shifting of +7.5 deg. Tr1Y/RConn1 -- Voltage Measurement/LConn1
  Three-Level Bridge  12Y/LConn1 -- Zigzag transformer Phase-Shifting of -7.5 deg. Tr2Y/RConn1 -- Voltage Measurement1/LConn1
  Three-Level Bridge 2D/LConn1 -- Zigzag transformer Phase-Shifting of -7.5 deg. Tr1Y2/RConn1 -- Voltage Measurement3/LConn1
  Imes_SE/LConn3 -- Breaker/RConn3 -- C1/RConn1
  "B1 "/RConn1 -- Imes_SE/LConn2 -- Breaker/RConn2
  Breaker/LConn3 -- Zigzag transformer Phase-Shifting of +7.5 deg. Tr1Y/LConn3 -- "C2 "/RConn1
  Breaker/LConn2 -- Zigzag transformer Phase-Shifting of +7.5 deg. Tr1Y/LConn2 -- "B2 "/RConn1
  Zigzag transformer Phase-Shifting of +7.5 deg. Tr1Y/LConn1 -- Breaker/LConn1 -- "A2 "/RConn1
  Three-Level Bridge  1Y/LConn3 -- Zigzag transformer Phase-Shifting of +7.5 deg. Tr1Y/RConn3
  Zigzag transformer Phase-Shifting of +7.5 deg. Tr1Y/RConn2 -- Three-Level Bridge  1Y/LConn2
  Three-Level Bridge  1D/LConn2 -- Zigzag transformer Phase-Shifting of +7.5 deg. Tr1Y1/RConn2 -- Voltage Measurement2/LConn2
  Three-Level Bridge  1D/LConn3 -- Zigzag transformer Phase-Shifting of +7.5 deg. Tr1Y1/RConn3
  Zigzag transformer Phase-Shifting of -7.5 deg. Tr2Y/RConn2 -- Three-Level Bridge  12Y/LConn2
  Three-Level Bridge  12Y/LConn3 -- Zigzag transformer Phase-Shifting of -7.5 deg. Tr2Y/RConn3
  Three-Level Bridge 2D/LConn2 -- Zigzag transformer Phase-Shifting of -7.5 deg. Tr1Y2/RConn2 -- Voltage Measurement3/LConn2
  Three-Level Bridge 2D/LConn3 -- Zigzag transformer Phase-Shifting of -7.5 deg. Tr1Y2/RConn3
